simulink subsystem "MySupercapacitor"  (R2023b)
settings: Solver=VariableStepAuto  StartTime=0.0  StopTime=10.0  RelTol=1e-3
values from neighbouring files (symbols this model uses):
  C0 = 623    [init_variables.m]
  C2 = 2100    [init_variables.m]
  Cv = 172    [init_variables.m]
  Np_sc = 5    [init_variables.m]
  Ns_sc = 9    [init_variables.m]
  R1 = 0.36e-03    (= 0.00036)    [init_variables.m]
  R2 = 1.92    [init_variables.m]
settings Model: Creator=xyh53  LastModifiedBy=xyh53

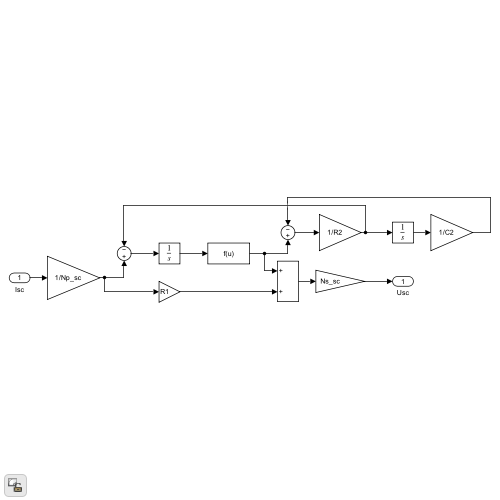
[thumbnail: Simulink's stored preview of the top-level diagram]
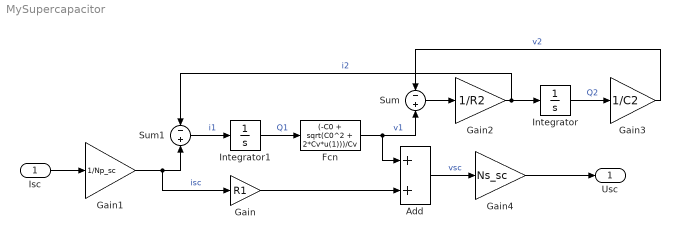
== system MySupercapacitor ==
  Isc : Inport
  Add : Sum
  Fcn : Fcn  Expr=(-C0 + sqrt(C0^2 + 2*Cv*u(1)))/Cv
  Gain : Gain  Gain=R1
  Gain1 : Gain  Gain=1/Np_sc
  Gain2 : Gain  Gain=1/R2
  Gain3 : Gain  Gain=1/C2
  Gain4 : Gain  Gain=Ns_sc
  Integrator : Integrator
  Integrator1 : Integrator
  Sum : Sum  Inputs=-+
  Sum1 : Sum  Inputs=-+
  Usc : Outport
  wires:
  Fcn/1 -> Add/1, Sum/2  "v1"
  Isc/1 -> Gain1/1
  Sum1/1 -> Integrator1/1  "i1"
  Gain1/1 -> Sum1/2, Gain/1  "isc"
  Integrator1/1 -> Fcn/1  "Q1"
  Gain/1 -> Add/2
  Sum/1 -> Gain2/1
  Add/1 -> Gain4/1  "vsc"
  Gain2/1 -> Sum1/1, Integrator/1  "i2"
  Gain4/1 -> Usc/1
  Integrator/1 -> Gain3/1  "Q2"
  Gain3/1 -> Sum/1  "v2"
